simulink model "final"  (R2013a)
settings: Solver=ode45  StartTime=0.0  StopTime=1  RelTol=1e-3
libraries: powerlib x34, simulink x1
settings Model: Creator=shridhana  LastModifiedBy=shridhana

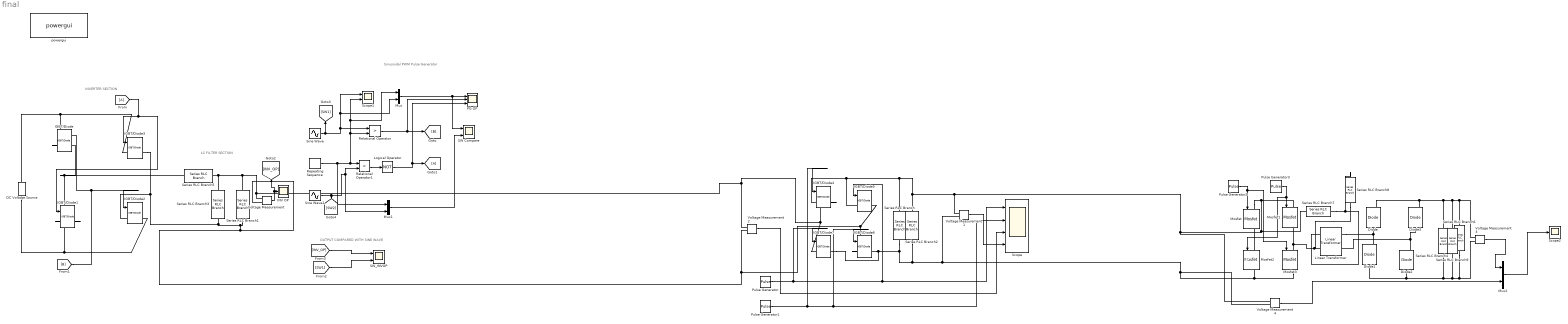
== system final ==
  note: OUTPUT COMPARED WITH
      | SINE WAVE
  note: INVERTER SECTION
  note: Sinusoidal PWM Pulse Generator
  note: LC FILTER SECTION
  note: z
  DC Voltage Source : powerlib/Electrical Sources/DC Voltage Source  Amplitude=230  Measurements=None
  Diode{,1..3} (4 alike) : powerlib/Power Electronics/Diode  Ron=0.001  Lon=0  Vf=0.8  IC=0  UseSnubber=off  Rs=500  Cs=250e-9  Measurements=on
  IGBT/Diode{,1..7} (8 alike) : powerlib/Power Electronics/IGBT//Diode  Ron=1e-3  Rs=1e5  Cs=inf  Measurements=on
  INV OP : Scope
      settings: TimeRange=1  YMin=-300  YMax=300  SaveName=ScopeData2
  Linear Transformer : powerlib/Elements/Linear Transformer  LConnTagsString=a|b  RConnTagsString=A|B  UNITS=SI  NominalPower=[8e3 20000 ]  winding1=[100 0.00025 0]  winding2=[486 0.0004 0]  ThreeWindings=off  winding3=[3.15e+05 24806 7.8961]  RmLm=[1000 21.518e-6]  Measurements=None  DataType=on
  Logical Operator : Logic  Operator=NOT  AllPortsSameDT=off  OutDataTypeStr=boolean
  Mosfet{,1..3} (4 alike) : powerlib/Power Electronics/Mosfet  Ron=2e-3  Lon=0  Rd=2e-3  Vfd=1  IC=0  Rs=1e5  Cs=inf  Measurements=on
  Mux : Mux  Inputs=2
  Mux1 : Mux  Inputs=2
  Mux2 : Mux  Inputs=2
  PG OP : Scope  NumInputPorts=3
      settings: YMin=-10~-5~-5  YMax=10~5~5
  Pulse Generator : DiscretePulseGenerator  PulseType=Time based  Amplitude=10  Period=20e-3  PulseWidth=5  PhaseDelay=2
  Pulse Generator1 : DiscretePulseGenerator  PulseType=Time based  Amplitude=10  Period=20e-3  PulseWidth=5  PhaseDelay=1
  Pulse Generator2 : DiscretePulseGenerator  PulseType=Time based  Amplitude=5  Period=50e-6  PulseWidth=50
  Pulse Generator3 : DiscretePulseGenerator  PulseType=Time based  Amplitude=5  Period=50e-6  PulseWidth=50  PhaseDelay=25e-6
  Relational Operator : RelationalOperator  Operator=>  OutDataTypeStr=boolean
  Relational Operator1 : RelationalOperator  Operator=>  OutDataTypeStr=boolean
  Repeating Sequence : simulink/Sources/Repeating Sequence  rep_seq_t=[0 0.5 1]*(1/1000)  rep_seq_y=[0 1 0]
  SW Compare : Scope  NumInputPorts=2
      settings: YMin=-10~-5  YMax=10~5  SaveName=ScopeData3
  SW_INVOP : Scope  NumInputPorts=2
      settings: YMin=-250~-0.8  YMax=250~0.8  SaveName=ScopeData4
  Scope : Scope  NumInputPorts=4
      settings: TimeRange=1.053745218223906  YMin=0~0~-100~-0  YMax=10~10~100~150  SaveName=ScopeData5
  Scope1 : Scope  NumInputPorts=2
      settings: YMin=-5~-5  YMax=5~5
  Scope2 : Scope
      settings: YMin=165  YMax=230  SaveName=ScopeData6  Decimation=20
  Series RLC Branch : powerlib/Elements/Series RLC Branch  LConnTagsString=__new0  RConnTagsString=__new0  BranchType=C  Resistance=10  Inductance=1e-4  SetiL0=off  InitialCurrent=0  Capacitance=435e-4  Setx0=off  InitialVoltage=0  Measurements=None
  Series RLC Branch1 : powerlib/Elements/Series RLC Branch  LConnTagsString=__new0  RConnTagsString=__new0  BranchType=R  Resistance=50  Inductance=40e-3  SetiL0=off  InitialCurrent=0  Capacitance=500e-3  Setx0=off  InitialVoltage=0  Measurements=None
  Series RLC Branch2 : powerlib/Elements/Series RLC Branch  LConnTagsString=__new0  RConnTagsString=__new0  BranchType=R  Resistance=130  Inductance=1e-4  SetiL0=off  InitialCurrent=0  Capacitance=1e-1  Setx0=off  InitialVoltage=0  Measurements=None
  Series RLC Branch3 : powerlib/Elements/Series RLC Branch  LConnTagsString=__new0  RConnTagsString=__new0  BranchType=C  Resistance=1  Inductance=40e-3  SetiL0=off  InitialCurrent=0  Capacitance=1.9e-4  Setx0=off  InitialVoltage=0  Measurements=None
  Series RLC Branch4 : powerlib/Elements/Series RLC Branch  LConnTagsString=__new0  RConnTagsString=__new0  BranchType=C  Resistance=1  Inductance=1e-3  SetiL0=off  InitialCurrent=0  Capacitance=6.2e-6  Setx0=off  InitialVoltage=0  Measurements=Branch voltage
  Series RLC Branch5 : powerlib/Elements/Series RLC Branch  LConnTagsString=__new0  RConnTagsString=__new0  BranchType=L  Resistance=1  Inductance=500e-4  SetiL0=off  InitialCurrent=0  Capacitance=500e-3  Setx0=off  InitialVoltage=0  Measurements=None
  Series RLC Branch6 : powerlib/Elements/Series RLC Branch  LConnTagsString=__new0  RConnTagsString=__new0  BranchType=R  Resistance=85.47  Inductance=1e-3  SetiL0=off  InitialCurrent=0  Capacitance=10e-6  Setx0=off  InitialVoltage=0  Measurements=Branch voltage
  Series RLC Branch7 : powerlib/Elements/Series RLC Branch  LConnTagsString=__new0  RConnTagsString=__new0  BranchType=LC  Resistance=100  Inductance=4.06e-6  SetiL0=off  InitialCurrent=0  Capacitance=0.52e-6  Setx0=off  InitialVoltage=0  Measurements=Branch voltage
  Series RLC Branch8 : powerlib/Elements/Series RLC Branch  LConnTagsString=__new0  RConnTagsString=__new0  BranchType=L  Resistance=100  Inductance=21.518e-6  SetiL0=off  InitialCurrent=0  Capacitance=10e-6  Setx0=off  InitialVoltage=0  Measurements=Branch voltage
  Series RLC Branch9 : powerlib/Elements/Series RLC Branch  LConnTagsString=__new0  RConnTagsString=__new0  BranchType=C  Resistance=1  Inductance=1e-3  SetiL0=off  InitialCurrent=0  Capacitance=6.2e-5  Setx0=off  InitialVoltage=0  Measurements=Branch voltage
  Sine Wave : Sin  Amplitude=0.8  Frequency=2*pi*50  SampleTime=0
  Sine Wave1 : Sin  Amplitude=0.8  Frequency=2*pi*50  Phase=pi  SampleTime=0
  Voltage Measurement{,1..4} (5 alike) : powerlib/Measurements/Voltage Measurement  PhasorSimulation=off  OutputType=Complex  PSBequivalent=0
  powergui : powerlib/powergui  Priority=1  SimulationMode=Continuous  SolverType=Tustin  SampleTime=1e-8  frequency=60  SPID=off  DisableSnubberDevices=off  DisableRonSwitches=off  DisableVfSwitches=off  SwTol=0  Interpol=off  DisplayEquations=off  frequencyindice=0  Pbase=100e6  ErrMax=1e-4  Iterations=50  UnitsV=kV  UnitsW=MW  FunctionMessages=off  echomessages=off  HookPort=off  EnableUseOfTLC=off  x0status=blocks  RestoreLinks=warning  ResistiveCurrentMeasurement=off  Frange=[0:2:500]  Ylog=off  Xlog=on  ShowGrid=off  save=off  variable=ZData  structure=0  ZoomFFT=off  StartTime=0.0  cycles=1  DisplayStyle=1  fundamental=60  FreqAxis=off  MaxFrequency=1000  frequencyindicesteady=1  RmsSteady=1  display=off  Ts=100  methode=off
  wires:
  [A] -> IGBT/Diode1/1, IGBT/Diode3/1
  [B] -> IGBT/Diode2/1, IGBT/Diode/1
  Sine Wave/1 -> [SW1], Relational Operator/1, Mux/2, Scope1/1
  Relational Operator/1 -> PG OP/2, [B]
  Mux/1 -> PG OP/1, SW Compare/1
  Repeating Sequence/1 -> Mux1/1, Relational Operator/2, Mux/1, Scope1/2, Relational Operator1/1
  Sine Wave1/1 -> [SW2], Mux1/2, Relational Operator1/2
  Relational Operator1/1 -> Logical Operator/1
  Logical Operator/1 -> PG OP/3, [A]
  Mux1/1 -> SW Compare/2
  Voltage Measurement/1 -> [INV_OP], INV OP/1
  [INV_OP] -> SW_INVOP/1
  [SW1] -> SW_INVOP/2
  Pulse Generator1/1 -> Scope/2, IGBT/Diode6/1, IGBT/Diode4/1
  Pulse Generator/1 -> Scope/1, IGBT/Diode5/1, IGBT/Diode7/1
  Voltage Measurement2/1 -> Scope/3
  Voltage Measurement1/1 -> Scope/4
  ? -> ?
  Voltage Measurement3/1 -> Mux2/1
  Pulse Generator2/1 -> Mosfet/1, Mosfet3/1
  Pulse Generator3/1 -> Mosfet2/1, Mosfet1/1
  Voltage Measurement4/1 -> Mux2/2
  Mux2/1 -> Scope2/1
  connections:
  IGBT/Diode3/LConn1 -- DC Voltage Source/RConn1 -- IGBT/Diode/LConn1
  IGBT/Diode2/RConn1 -- DC Voltage Source/LConn1 -- IGBT/Diode1/RConn1
  IGBT/Diode1/LConn1 -- Series RLC Branch5/LConn1 -- IGBT/Diode/RConn1
  IGBT/Diode7/LConn1 -- Series RLC Branch5/RConn1 -- Series RLC Branch3/LConn1 -- Series RLC Branch1/RConn1 -- Voltage Measurement/LConn1 -- Voltage Measurement2/LConn1 -- IGBT/Diode4/RConn1
  IGBT/Diode5/RConn1 -- Series RLC Branch1/LConn1 -- IGBT/Diode3/RConn1 -- IGBT/Diode2/LConn1 -- Series RLC Branch3/RConn1 -- Voltage Measurement/LConn2 -- Voltage Measurement2/LConn2 -- IGBT/Diode6/LConn1
  Mosfet1/RConn1 -- Mosfet3/LConn1 -- Linear Transformer/LConn2 -- Series RLC Branch8/RConn1
  Mosfet/LConn1 -- Mosfet1/LConn1 -- Series RLC Branch7/RConn1 -- Voltage Measurement4/LConn1 -- Series RLC Branch/LConn1 -- IGBT/Diode5/LConn1 -- IGBT/Diode4/LConn1 -- Series RLC Branch2/LConn1 -- Voltage Measurement1/LConn1
  Voltage Measurement4/LConn2 -- IGBT/Diode7/RConn1 -- IGBT/Diode6/RConn1 -- Series RLC Branch/RConn1 -- Series RLC Branch2/RConn1 -- Voltage Measurement1/LConn2 -- Mosfet3/RConn1 -- Mosfet2/RConn1
  Linear Transformer/RConn2 -- Diode2/RConn1 -- Diode3/LConn1
  Diode/LConn1 -- Linear Transformer/RConn1 -- Diode1/RConn1
  Voltage Measurement3/LConn2 -- Series RLC Branch6/RConn1 -- Series RLC Branch9/RConn1 -- Series RLC Branch4/RConn1 -- Diode2/LConn1 -- Diode1/LConn1
  Series RLC Branch4/LConn1 -- Series RLC Branch9/LConn1 -- Voltage Measurement3/LConn1 -- Series RLC Branch6/LConn1 -- Diode3/RConn1 -- Diode/RConn1
  Series RLC Branch8/LConn1 -- Linear Transformer/LConn1 -- Series RLC Branch7/LConn1
  Mosfet2/LConn1 -- Mosfet/RConn1
